simulink model "teht3"  (Simulink 7.4)
settings: Solver=ode45  StartTime=0.0  StopTime=10.0  RelTol=1e-3
libraries: fuzblock x1
settings Model: Creator=Leonardo  LastModifiedBy=Leonardo
settings DebuggingCC: SolverPrmCheckMsg=none

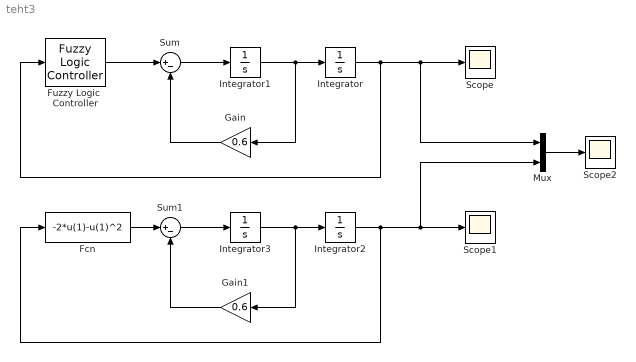
== system teht3 ==
  Fcn : Fcn  Expr=-2*u(1)-u(1)^2
  Fuzzy Logic  Controller : fuzblock/Fuzzy Logic  Controller  SystemSampleTime=-1  fis=fismat1
  Gain : Gain  Gain=0.6  ParameterDataType=fixdt(1, 16)  ParameterScaling=2^0  OutDataType=fixdt(1, 16)  OutScaling=2^0
  Gain1 : Gain  Gain=0.6  ParameterDataType=fixdt(1, 16)  ParameterScaling=2^0  OutDataType=fixdt(1, 16)  OutScaling=2^0
  Integrator : Integrator  InitialCondition=-0.2
  Integrator1 : Integrator  InitialCondition=0.5
  Integrator2 : Integrator  InitialCondition=-0.2
  Integrator3 : Integrator  InitialCondition=0.5
  Mux : Mux  Inputs=2
  Scope : Scope
  Scope1 : Scope
  Scope2 : Scope
      settings: SaveName=ScopeData2
  Sum : Sum  Inputs=|+-  OutDataType=fixdt(1, 16)  OutScaling=2^0
  Sum1 : Sum  Inputs=|+-  OutDataType=fixdt(1, 16)  OutScaling=2^0
  wires:
  Fuzzy Logic  Controller/1 -> Sum/1
  Sum/1 -> Integrator1/1
  Integrator1/1 -> Integrator/1, Gain/1
  Gain/1 -> Sum/2
  Integrator/1 -> Fuzzy Logic  Controller/1, Scope/1, Mux/1
  Fcn/1 -> Sum1/1
  Sum1/1 -> Integrator3/1
  Integrator3/1 -> Integrator2/1, Gain1/1
  Gain1/1 -> Sum1/2
  Integrator2/1 -> Fcn/1, Scope1/1, Mux/2
  Mux/1 -> Scope2/1
